simulink model "flywheel_speed_ctrl_with_load_observer"  (R2020a)
settings: Solver=ode23tb  StartTime=0.0  StopTime=simulation_length  MaxStep=ts
undefined symbols (not defined in the file): A, Aed, B, Bed, C, Ce, E, ki, kp, Led, Tc, ts
settings Model: SimulationMode=accelerator  Creator=dbagn  LastModifiedBy=dbagn
settings DataIOCC: SaveTime=off  ReturnWorkspaceOutputs=off
settings SFSimCC: SimCustomHeaderCode="#include \"sfbctrl.h\""  SimUserSources=src/sfbctrl.c  SimUserIncludeDirs=include  SimParseCustomCode=off

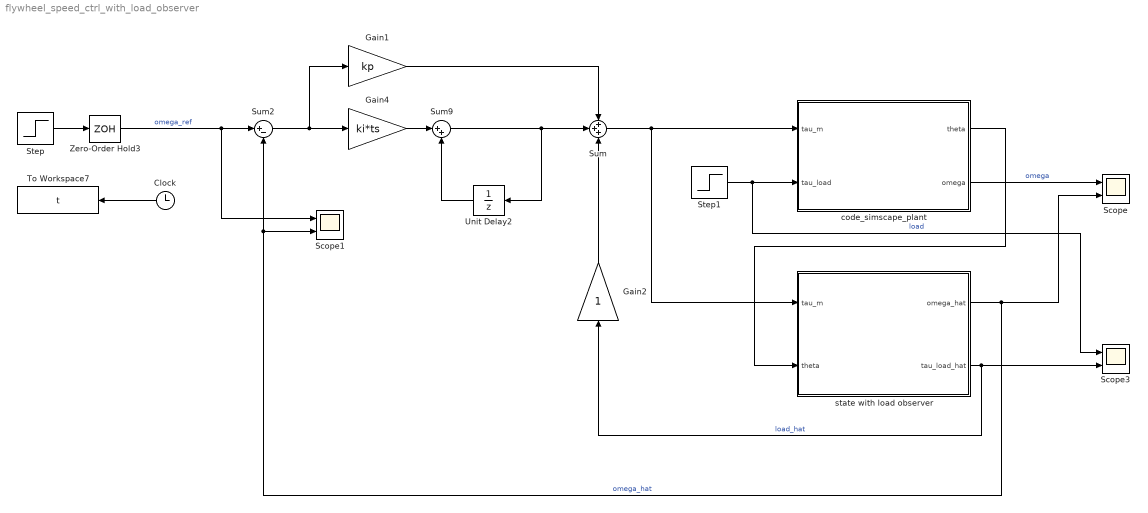
== system flywheel_speed_ctrl_with_load_observer ==
  Clock : Clock
  Gain1 : Gain  Gain=kp
  Gain2 : Gain
  Gain4 : Gain  Gain=ki*ts
  Scope : Scope  NumInputPorts=2
  Scope1 : Scope  NumInputPorts=2
  Scope3 : Scope  NumInputPorts=2
  Step : Step  Time=0.2  SampleTime=0
  Step1 : Step  After=25  SampleTime=0
  Sum : Sum  Inputs=+++
  Sum2 : Sum  Inputs=|+-
  Sum9 : Sum  Inputs=|++
  To Workspace7 : ToWorkspace  VariableName=t  SampleTime=Tc
      settings: MaxDataPoints=Nc
  Unit Delay2 : UnitDelay  SampleTime=ts  HasFrameUpgradeWarning=on
  Zero-Order Hold3 : ZeroOrderHold  SampleTime=ts
  "code_simscape_plant " : Subsystem
  state with load observer : Subsystem
  wires:
  Clock/1 -> To Workspace7/1
  Zero-Order Hold3/1 -> Scope1/1, Sum2/1  "omega_ref"
  Unit Delay2/1 -> Sum9/2
  Step/1 -> Zero-Order Hold3/1
  Gain4/1 -> Sum9/1
  Sum9/1 -> Unit Delay2/1, Sum/2
  Sum2/1 -> Gain1/1, Gain4/1
  Gain1/1 -> Sum/1
  Sum/1 -> state with load observer/1(tau_m), "code_simscape_plant "/1(tau_m)
  Step1/1 -> "code_simscape_plant "/2(tau_load), Scope3/1  "load"
  "code_simscape_plant "/1(theta) -> state with load observer/2(theta)
  "code_simscape_plant "/2(omega) -> Scope/1  "omega"
  state with load observer/1(omega_hat) -> Scope/2, Scope1/2, Sum2/2  "omega_hat"
  state with load observer/2(tau_load_hat) -> Gain2/1, Scope3/2  "load_hat"
  Gain2/1 -> Sum/3

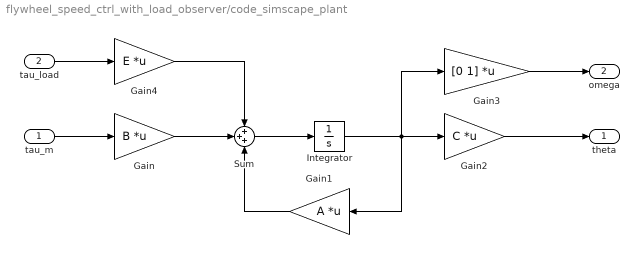
== system flywheel_speed_ctrl_with_load_observer/code_simscape_plant  ==
  tau_m : Inport
  tau_load : Inport  Port=2
  Gain : Gain  Gain=B  Multiplication=Matrix(K*u)
  Gain1 : Gain  Gain=A  Multiplication=Matrix(K*u)
  Gain2 : Gain  Gain=C  Multiplication=Matrix(K*u)
  Gain3 : Gain  Gain=[0 1]  Multiplication=Matrix(K*u)
  Gain4 : Gain  Gain=E  Multiplication=Matrix(K*u)
  Integrator : Integrator
  Sum : Sum  Inputs=+++
  theta : Outport
  omega : Outport  Port=2
  wires:
  Sum/1 -> Integrator/1
  Integrator/1 -> Gain3/1, Gain2/1, Gain1/1
  Gain2/1 -> theta/1
  tau_m/1 -> Gain/1
  Gain3/1 -> omega/1
  tau_load/1 -> Gain4/1
  Gain/1 -> Sum/2
  Gain1/1 -> Sum/3
  Gain4/1 -> Sum/1

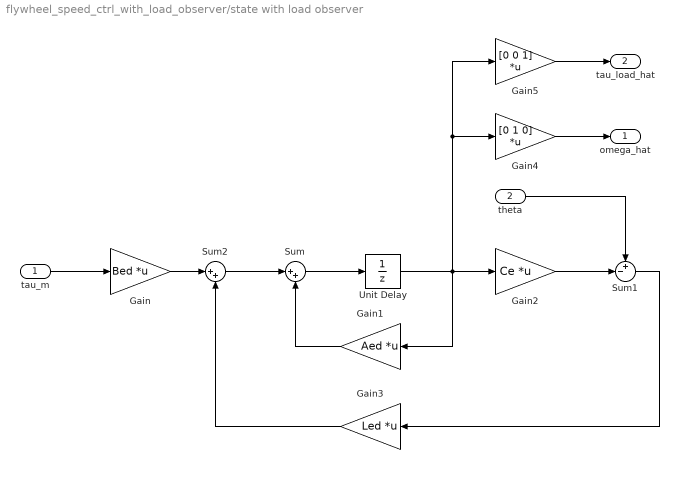
== system flywheel_speed_ctrl_with_load_observer/state with load observer ==
  tau_m : Inport
  theta : Inport  Port=2
  Gain : Gain  Gain=Bed  Multiplication=Matrix(K*u)
  Gain1 : Gain  Gain=Aed  Multiplication=Matrix(K*u)
  Gain2 : Gain  Gain=Ce  Multiplication=Matrix(K*u)
  Gain3 : Gain  Gain=Led  Multiplication=Matrix(K*u)
  Gain4 : Gain  Gain=[0 1 0]  Multiplication=Matrix(K*u)
  Gain5 : Gain  Gain=[0 0 1]  Multiplication=Matrix(K*u)
  Sum : Sum  Inputs=|++
  Sum1 : Sum  Inputs=+-|
  Sum2 : Sum  Inputs=|++
  Unit Delay : UnitDelay  SampleTime=ts  HasFrameUpgradeWarning=on
  omega_hat : Outport
  tau_load_hat : Outport  Port=2
  wires:
  Sum/1 -> Unit Delay/1
  tau_m/1 -> Gain/1
  Gain1/1 -> Sum/2
  Gain2/1 -> Sum1/2
  theta/1 -> Sum1/1
  Gain/1 -> Sum2/1
  Sum2/1 -> Sum/1
  Sum1/1 -> Gain3/1
  Gain3/1 -> Sum2/2
  Unit Delay/1 -> Gain5/1, Gain4/1, Gain2/1, Gain1/1
  Gain4/1 -> omega_hat/1
  Gain5/1 -> tau_load_hat/1
